simulink model "sistema_non_linearizzato_condizioni_inziali"  (R2025b)
settings: Solver=VariableStepAuto  StartTime=0.0  StopTime=5  RelTol=1e-3
values from neighbouring files (symbols this model uses):
  C = [0 1]    [scaldatore.m]
  ue = (h_r*A_r)*(x_e(1) - x_e(2))*(1 + k*x_e(1))    [scaldatore.m]
  x2_e = 27.1911    [scaldatore.m]
  x_e = [x1_e;x2_e]    [scaldatore.m]
libraries: cstblocks x1
settings Model: Creator=s0001117122  LastModifiedBy=doddo

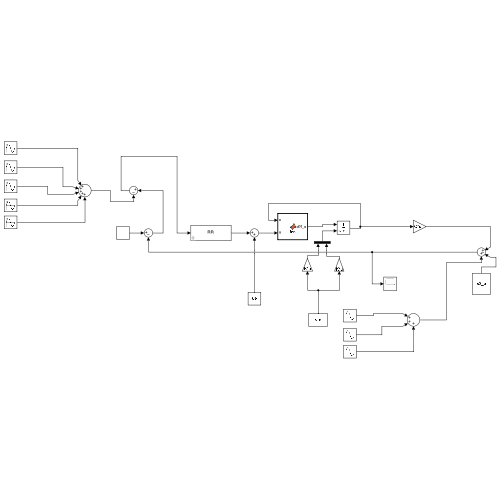
[thumbnail: Simulink's stored preview of the top-level diagram]
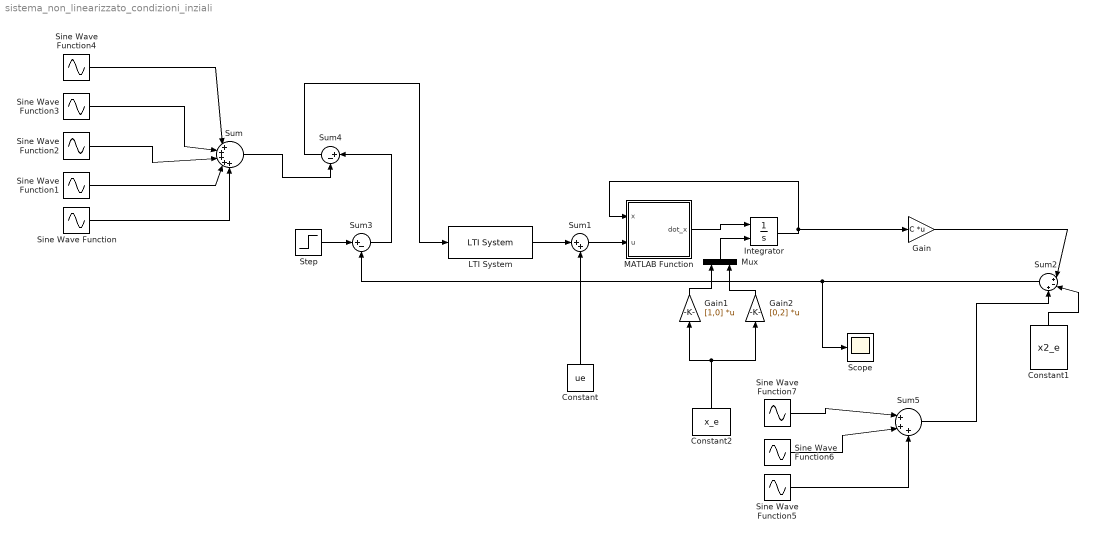
== system sistema_non_linearizzato_condizioni_inziali ==
  Constant : Constant  Value=ue
  Constant1 : Constant  Value=x2_e
  Constant2 : Constant  Value=x_e
  Gain : Gain  Gain=C  Multiplication=Matrix(K*u)
  Gain1 : Gain  Gain=[1,0]  Multiplication=Matrix(K*u)
  Gain2 : Gain  Gain=[0,2]  Multiplication=Matrix(K*u)
  Integrator : Integrator  InitialConditionSource=external  InitialCondition=[300;90]
  LTI System : cstblocks/LTI System  sys=RR  IC=[]  PadeOrder=0
  MATLAB Function : MATLAB Function  TreatAsAtomicUnit=on
  Mux : Mux  Inputs=2
  Scope : Scope
      settings: ActiveDisplayYMinimum=9.3033948130674382  ActiveDisplayYMaximum=23.663994847681209
  Sine Wave Function : Sin  Amplitude=0.5  Frequency=10^5  SampleTime=0
  Sine Wave Function1 : Sin  Amplitude=0.5  Frequency=10^5*2  SampleTime=0
  Sine Wave Function2 : Sin  Amplitude=0.5  Frequency=10^5*3  SampleTime=0
  Sine Wave Function3 : Sin  Amplitude=0.5  Frequency=10^5*4  SampleTime=0
  Sine Wave Function4 : Sin  Amplitude=0.5  Frequency=10^5*5  SampleTime=0
  Sine Wave Function5 : Sin  Amplitude=0.5  Frequency=0.05*3  SampleTime=0
  Sine Wave Function6 : Sin  Amplitude=2  Frequency=0.05*2  SampleTime=0
  Sine Wave Function7 : Sin  Amplitude=2  Frequency=0.05  SampleTime=0
  Step : Step  Time=0  After=15  SampleTime=0
  Sum : Sum  Inputs=|+++++
  Sum1 : Sum  Inputs=|++
  Sum2 : Sum  Inputs=|+-+
  Sum3 : Sum  Inputs=|+-
  Sum4 : Sum  Inputs=|+-
  Sum5 : Sum  Inputs=|+++
  wires:
  MATLAB Function/1(dot_x) -> Integrator/1
  Integrator/1 -> Gain/1, MATLAB Function/1(x)
  Gain/1 -> Sum2/1
  Constant1/1 -> Sum2/2
  Constant/1 -> Sum1/2
  LTI System/1 -> Sum1/1
  Sum2/1 -> Scope/1, Sum3/2
  Sum1/1 -> MATLAB Function/2(u)
  Step/1 -> Sum3/1
  Sum3/1 -> Sum4/1
  Sine Wave Function/1 -> Sum/5
  Sine Wave Function1/1 -> Sum/4
  Sine Wave Function2/1 -> Sum/3
  Sine Wave Function3/1 -> Sum/2
  Sine Wave Function4/1 -> Sum/1
  Sum/1 -> Sum4/2
  Sum4/1 -> LTI System/1
  Sine Wave Function7/1 -> Sum5/1
  Sine Wave Function6/1 -> Sum5/2
  Sine Wave Function5/1 -> Sum5/3
  Sum5/1 -> Sum2/3
  Constant2/1 -> Gain2/1, Gain1/1
  Gain2/1 -> Mux/2
  Gain1/1 -> Mux/1
  Mux/1 -> Integrator/2

== matlab function sistema_non_linearizzato_condizioni_inziali/MATLAB Function ==
  data: x input; dot_x output; u input
function dot_x = fcn(x, u)

h_r = 40; % [W/(m^2 C°)] Coefficiente di convezione tra riscaldatore e aria
A_r=0.13; % [m^2] Area di scambio termico tra riscaldatore e aria
c_r=858.8; % [J/(kg C°)] Calore specifico del riscaldatore
c_a=1010; % [J/(kg C°)] Calore specifico dell'aria
m_r=1.849; % [kg] Massa del riscaldatore
m_a=0.1041; % [kg] Massa dell'aria
mm_a=0.2; % [kg/s] Portata massica dell’aria
T_in=23; % [C°] Temperatura dell’aria in ingresso (ambiente a temperatura costante)
k=2.5*1e-3; % [1/C°] Coefficiente di variazione della resistenza con la temperatura

dot_x = zeros(2,1);

dot_x(1) =  (  h_r * A_r * (x(2) - x(1)) + u / (1 + k * x(1)) ) / (m_r * c_r);

dot_x(2) = (mm_a * c_a * (T_in -x(2)) + h_r * A_r * (x(1)-x(2)))/(m_a*c_a);
